simulink model "Lab2_single_loop_controller_student_manual"  (R2025a)
settings: Solver=FixedStepAuto  StartTime=0.0  StopTime=20  FixedStep=0.0002  MaxStep=0.01  RelTol=1e-3
values from neighbouring files (symbols this model uses):
  g = 9.81    [Lab2_before_after.m]    (also in Lab2_cascade_controller_experimentation.m; Lab2_experimentation.m; Lab2_manual_params_student.m; Lab2_manual_simulate_controller.m)
  gravity_compensation_mode = 1    [Lab2_cascade_controller_experimentation.m]    (also in Lab2_manual_params_student.m; Lab2_manual_simulate_controller.m = params.gravity_mode; Lab2_params_student.m)
  init_angle = 0    [Lab2_cascade_controller_experimentation.m]    (also in Lab2_experimentation.m; Lab2_manual_params_student.m; Lab2_manual_simulate_controller.m = params.init)
  J = 58.559e-6    (= 5.8559e-05)    [Lab2_before_after.m]    (also in Lab2_cascade_controller_experimentation.m; Lab2_experimentation.m; Lab2_manual_params_student.m; Lab2_manual_simulate_controller.m)
  kd = 0.1111    [Lab2_cascade_controller_experimentation.m]    (also in Lab2_manual_PID_comparison.m = ifthen(isfield(S_meta.params, 'kd'), S_meta.params.kd, 0); Lab2_manual_params_student.m = 0.445677002796; Lab2_manual_simulate_controller.m = params.kd; Lab2_params_student.m = 0)
  ke = 52.8e-3    (= 0.0528)    [Lab2_before_after.m]    (also in Lab2_cascade_controller_experimentation.m; Lab2_experimentation.m; Lab2_manual_params_student.m; Lab2_manual_simulate_controller.m)
  ki = 0    [Lab2_cascade_controller_experimentation.m]    (also in Lab2_manual_PID_comparison.m = ifthen(isfield(S_meta.params, 'ki'), S_meta.params.ki, 0); Lab2_manual_params_student.m = 0.135074981664; Lab2_manual_simulate_controller.m = params.ki; Lab2_params_student.m)
  kp = 0.071701766537834    (= 0.0717017665378)    [Lab2_cascade_controller_experimentation.m]    (also in Lab2_manual_PID_comparison.m = S_meta.params.kp; Lab2_manual_params_student.m = 0.633530931368; Lab2_manual_simulate_controller.m = params.kp; Lab2_params_student.m = 0)
  kt = 50.6e-3    (= 0.0506)    [Lab2_before_after.m]    (also in Lab2_cascade_controller_experimentation.m; Lab2_experimentation.m; Lab2_manual_params_student.m; Lab2_manual_simulate_controller.m)
  L = 0.1    [Lab2_before_after.m]    (also in Lab2_cascade_controller_experimentation.m; Lab2_cascade_lab_setup.m = length(data.time); Lab2_experimentation.m; Lab2_manual_params_student.m)
  Lm = 2.8544e-3    (= 0.0028544)    [Lab2_before_after.m]    (also in Lab2_cascade_controller_experimentation.m; Lab2_experimentation.m; Lab2_manual_params_student.m; Lab2_manual_simulate_controller.m)
  method_pid = 2    [Lab2_cascade_controller_experimentation.m]    (also in Lab2_manual_params_student.m; Lab2_manual_simulate_controller.m = params.method; Lab2_params_student.m = 1)
  mp = 0.05    [Lab2_before_after.m]    (also in Lab2_cascade_controller_experimentation.m; Lab2_experimentation.m; Lab2_manual_params_student.m; Lab2_manual_simulate_controller.m)
  N = 100    [Lab2_cascade_controller_experimentation.m]    (also in Lab2_manual_lab_setup.m; Lab2_manual_params_student.m = 1389.45650583; Lab2_manual_simulate_controller.m = params.N)
  R = 3.3133    [Lab2_before_after.m]    (also in Lab2_cascade_controller_experimentation.m; Lab2_experimentation.m; Lab2_manual_params_student.m; Lab2_manual_simulate_controller.m)
  ref_angle = 180    [Lab2_cascade_controller_experimentation.m]    (also in Lab2_manual_params_student.m; Lab2_params_student.m)
  s = tf('s')    [Lab2_manual_lab_setup.m]    (also in Lab2_pole_zero_plot.m; Labs2_tuner.m)
  T = Lm/Rm    (= 0.000861497600579)    [Lab2_cascade_controller_experimentation.m]    (also in Lab2_cascade_lab_setup.m = table(data.time, data.position_loop.position_ref, data.posit; Lab2_experimentation.m; Lab2_manual_params_student.m; Lab2_manual_simulate_controller.m)
  Y = fft(sig - mean(sig))    [Lab2_cascade_lab_setup.m]
undefined symbols (not defined in the file or in its folder): X, Z
libraries: sm_lib x14, nesl_utility x4, slpidlib x2
(part 1 of 2)
settings Model: Creator=User  LastModifiedBy=User
settings RTWCC: GPUComputeCapability=3.5

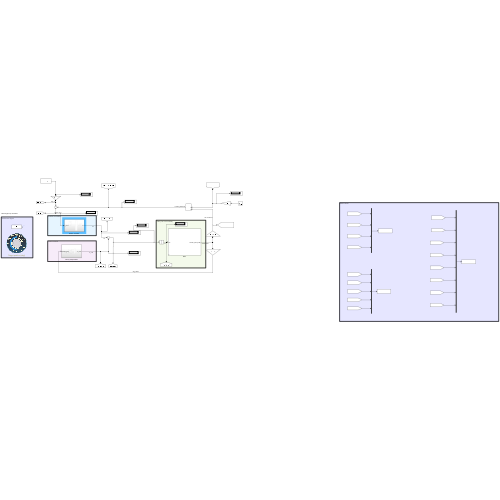
[thumbnail: Simulink's stored preview of the top-level diagram]
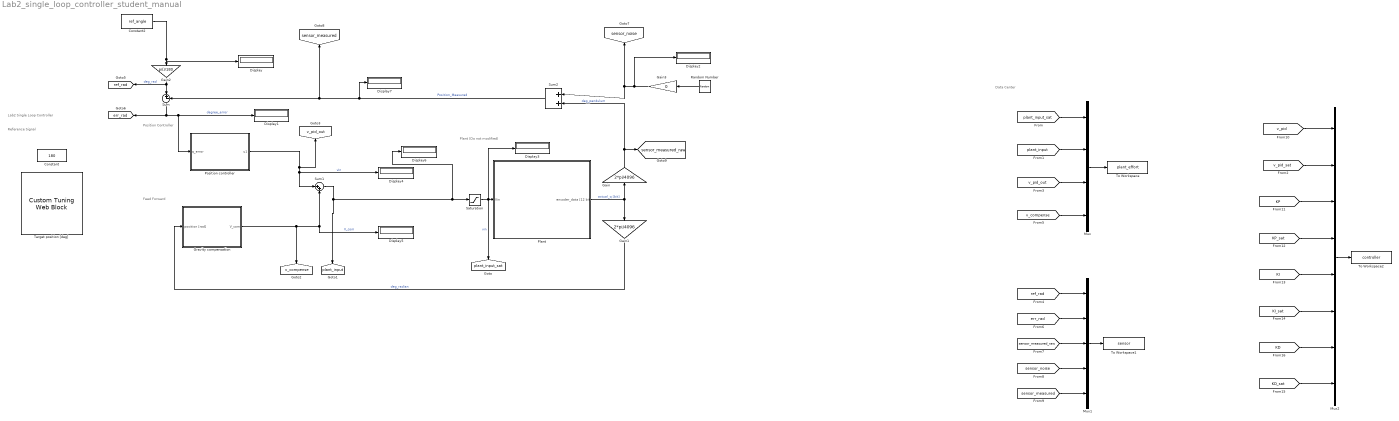
== system Lab2_single_loop_controller_student_manual ==
  note: Lab2 Single Loop Controller
  note: Plant (Do not modified)
  note: Feed Forward
  note: Position Controller
  note: Reference Signal
  note: Data Center
  Constant : Constant  Value=180  SampleTime=-1
  Constant2 : Constant  Value=ref_angle
  Display{,1..7} (8 alike) : Display
  Gain : Gain  Gain=2*pi/4096
  Gain1 : Gain  Gain=2*pi/4096
  Gain2 : Gain  Gain=pi()/180
  Gain3 : Gain  Gain=0
  Gravity compensation : Subsystem
  Mux : Mux
  Mux1 : Mux  Inputs=5
  Mux2 : Mux  Inputs=8
  Plant : Subsystem  mask{init_q=init_angle}
      mask prompts: init_q "Initial angle of pendulum [deg]"
  Position controller : Subsystem
  Random Number : RandomNumber  SampleTime=0.1
  Saturation : Saturate  UpperLimit=12  LowerLimit=-12
  Sum : Sum  Inputs=|+-
  Sum1 : Sum  Inputs=|++
  Sum2 : Sum  Inputs=|++
  Target position [deg] : CustomTuningWebBlock  LabelPosition=Hide  ShowInitialText=on  Configuration="{\"components\":[{\"name\":\"CircularScaleComponent\",\"settings\":{\"bounds\":{\"max\":360,\"min\":0,\"tickInterval\":30},\"direction\":\"cw\",\"flipLimits\":0,\"innerRadius\":0.6636618227670849,\"internalTickHeightScaleFactor\":1,\"labelColor\":[255,255,200],\"labelFont\":{\"font\":\"Arial\",\"fontSize\":12},\"labelRadius\":0.79,\"labelTransparency\":1,\"minorTickHeightScaleFactor\":0.2,\"needleImage\":{\"size\":[150,150],\"src\":\"data:image\\/svg+xml;base64,PD94bWwgdmVyc2lvbj0iMS4wIiBlbmNvZGluZz0idXRmLTgiPz4NCjwhLS0gR2VuZXJhdG9yOiBBZG9iZSBJbGx1c3RyYXRvciAyNS4yLjMsIFNWRyBFeHBvcnQgUGx1Zy1JbiAuIFNWRyBWZXJzaW9uOiA2LjAwIEJ1aWxkIDApICAtLT4NCjxzdmcgdmVyc2lvbj0iMS4xIiBpZD0iTGF5ZXJfMSIgeG1sbnM9Imh0dHA6Ly93d3cudzMub3JnLzIwMDAvc3ZnIiB4bWxuczp4bGluaz0iaHR0cDovL3d3dy53My5vcmcvMTk5OS94bGluayIgeD0iMHB4IiB5PSIwcHgiDQoJIHZpZXdCb3g9IjAgMCAxNTIgMTUyIiBzdHlsZT0iZW5hYmxl ...(+37472 chars)\"},\"needleOffset\":[0,0],\"needleOrientation\":-45,\"needleRotation\":90,\"needleSize\":{\"height\":0.44,\"width\":0.44},\"outerRadius\":0.5053386200069245,\"position\":[0,0,1,1],\"referencePoint\":\"auto\",\"scaleAngle\":360,\"scaleAngleOffset\":90,\"scaleColors\":[],\"scaleColorsSize\":0.2,\"scaleDirection\":\"CW\",\"scalePosition\":[0,0,1,1],\"showLabels\":1,\"showMinorTicks\":1,\"showSpanLine\":true,\"showTicks\":1,\"tickColor\":[252,252,197],\"tickTransparency\":1,\"valueBarColor\":[0,114,189],\"valueBarPosition\":[0,0,1,1],\"valueBarSize\":0.2,\"valueBarTransparency\":1}},{\"name\":\"BackgroundImageComponent\",\"settings\":{\"image\":{\"size\":[385,373],\"src\":\"data:image\\/svg+xml;base64,PD94bWwgdmVyc2lvbj0iMS4wIiBlbmNvZGluZz0idXRmLTgiPz4NCjwhLS0gR2VuZXJhdG9yOiBBZG9iZSBJbGx1c3RyYXRvciAyNS4wLjAsIFNWRyBFeHBvcnQgUGx1Zy1JbiAuIFNWRyBWZXJzaW9uOiA2LjAwIEJ1aWxkIDApICAtLT4NCjxzdmcgdmVyc2lvbj0iMS4xIg0KCSBpZD0iTGF5ZXJfMl8xXyIgeG1sbnM6Y2M9Imh0dHA6Ly9jcmVhdGl2ZWNvbW1vbnMub3JnL25zIyIgeG1sbnM6ZGM9Imh0dHA6Ly9wdXJsLm9yZy9kYy9lbGVtZW50cy8xLjEvIiB4bWxuczppbmtzY2FwZT0iaHR0cDovL3d3dy5pbmtzY2FwZS5vcmcv ...(+4184 chars)\",\"srcOrientation\":\"horizontal\"},\"position\":[0,0,1,1],\"scaleMode\":\"0\"}},{\"name\":\"ForegroundImageComponent\",\"settings\":{\"image\":{\"size\":[0,0],\"src\":\"default\",\"srcOrientation\":[]},\"isForeground\":1,\"position\":[0,0,1,1],\"scaleMode\":\"0\"}}],\"derived\":{\"blockParameters\":{\"ForegroundColor\":[0.9882352941176471,0.9882352941176471,0.7725490196078432],\"Limits\":{\"Max\":360,\"Min\":0,\"Ticks\":30},\"ScaleColors\":[],\"ScaleDirection\":\"Clockwise\",\"ScaleMax\":360,\"ScaleMin\":0,\"TickInterval\":30,\"fixedAspectRatio\":\"off\"}},\"settings\":{\"BindingType\":\"param\",\"aspectRatio\":1,\"backgroundColor\":[0,0,0,\"1\"],\"backgroundOffset\":1,\"backgroundOpacity\":1,\"direction\":\"cw\",\"fixedAspectRatio\":\"off\",\"flipLimits\":0,\"foregroundColor\":[252,252,196],\"orientation\":\"horizontal\",\"showBackgroundColor\":false,\"value\":0,\"version\":\"R2023a\"},\"type\":\"CircularGauge\"}"
  To Workspace : ToWorkspace  VariableName=plant_effort  SaveFormat=Timeseries  SampleTime=-1
  To Workspace1 : ToWorkspace  VariableName=sensor  SaveFormat=Timeseries  SampleTime=-1
  To Workspace2 : ToWorkspace  VariableName=controller  SaveFormat=Timeseries  SampleTime=-1
  tag scope: err_rad=global, plant_input=global, plant_input_sat=global, ref_rad=global, sensor_measured=global, sensor_measured_raw=global, sensor_noise=global, v_compense=global, v_pid_out=global
  wires:
  Saturation/1 -> Display3/1, Plant/1(Vin), [plant_input_sat]  "vin"
  Plant/1(encoder_data [12 bit]) -> Gain1/1, Gain/1  "actual_q [bit]"
  Gain/1 -> [sensor_measured_raw], Sum2/2  "deg_pendulum"
  Gain1/1 -> Gravity compensation/1(position [rad])  "deg_radian"
  Gravity compensation/1(V_com) -> [v_compense], Display5/1, Sum1/2  "V_com"
  Mux/1 -> To Workspace/1
  [plant_input_sat] -> Mux/1
  [plant_input] -> Mux/2
  Constant2/1 -> Display/1, Gain2/1
  Position controller/1(u1) -> Display4/1, Sum1/1, [v_pid_out]  "vin"
  [v_pid_out] -> Mux/3
  Gain3/1 -> Display2/1, Sum2/1, [sensor_noise]
  Random Number/1 -> Gain3/1
  Sum2/1 -> Display7/1, [sensor_measured], Sum/2  "Position_Measured"
  Gain2/1 -> [ref_rad], Sum/1  "deg_rad"
  Sum/1 -> [err_rad], Position controller/1(q_error), Display1/1  "degree_error"
  [err_rad] -> Mux1/2
  [sensor_noise] -> Mux1/4
  [sensor_measured_raw] -> Mux1/3
  [ref_rad] -> Mux1/1
  Mux1/1 -> To Workspace1/1
  [sensor_measured] -> Mux1/5
  [v_compense] -> Mux/4
  Mux2/1 -> To Workspace2/1
  [v_pid_sat] -> Mux2/2
  [v_pid] -> Mux2/1
  [KP] -> Mux2/3
  [KP_sat] -> Mux2/4
  [KI] -> Mux2/5
  [KI_sat] -> Mux2/6
  [KD] -> Mux2/7
  [KD_sat] -> Mux2/8
  Sum1/1 -> [plant_input], Display6/1, Saturation/1
